simulink model "SistemaUrinario_Simulink"  (R2023a)
settings: Solver=ode15s  StartTime=0.0  StopTime=10.0  RelTol=1e-3
libraries: slpidlib x1
settings Model: Creator=maria  LastModifiedBy=maria
settings DataIOCC: ReturnWorkspaceOutputs=off  TimeSaveName=t
settings DebuggingCC: AlgebraicLoopMsg=none  ArtificialAlgebraicLoopMsg=none  MaxConsecutiveZCsMsg=none  ModelReferenceExtraNoncontSigs=none  OperatingPointInterfaceChecksumMismatchMsg=none

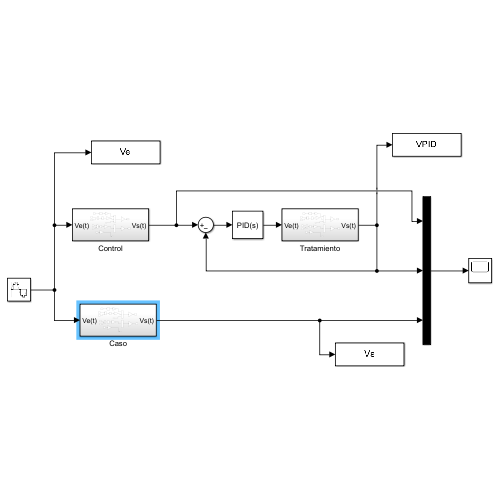
[thumbnail: Simulink's stored preview of the top-level diagram]
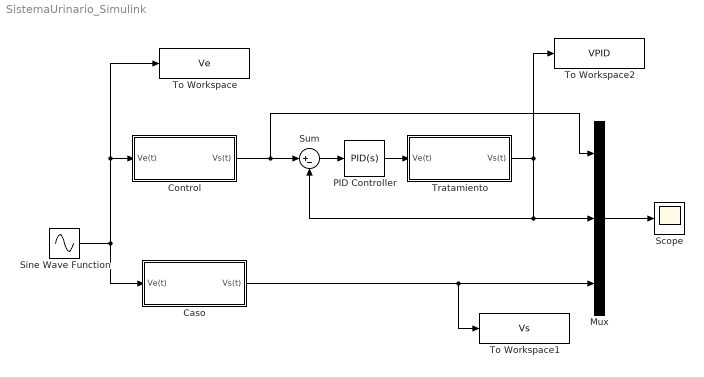
== system SistemaUrinario_Simulink ==
  Caso : Subsystem
  Control : Subsystem
  Mux : Mux  Inputs=3
  PID Controller : slpidlib/PID Controller  Controller=PID  Form=Parallel  TimeDomain=Continuous-time  UseExternalTs=off  SampleTime=-1  IntegratorMethod=Forward Euler  FilterMethod=Forward Euler  ControllerParametersSource=internal  P=8009847.10025754  I=198556446.374402  UseKiTs=off  D=40297.8764782752  N=86.9358796207791  UseFilter=on  TunerSelectOption=Transfer Function Based (PID Tuner App)  InitialConditionSource=internal  InitialConditionForIntegrator=0  InitialConditionForFilter=0  DifferentiatorICPrevScaledInput=0  ExternalReset=none  TrackingMode=off  Kt=1  LimitOutput=off  SatLimitsSource=internal  UpperSaturationLimit=inf  LowerSaturationLimit=-inf  LinearizeAsGain=on  AntiWindupMode=none  Kb=1  LimitIntegrator=off  UpperIntegratorSaturationLimit=inf  LowerIntegratorSaturationLimit=-inf  POutMin=[]  POutMax=[]  IOutMin=[]  IOutMax=[]  DOutMin=[]  DOutMax=[]  NOutMin=[]  NOutMax=[]  SumOutMin=[]  SumOutMax=[]  SaturationOutMin=[]  SaturationOutMax=[]  PParamMin=[]  PParamMax=[]  IParamMin=[]  IParamMax=[]  DParamMin=[]  DParamMax=[]  NParamMin=[]  NParamMax=[]  KbParamMin=[]  KbParamMax=[]  KtParamMin=[]  KtParamMax=[]  KbOutMin=[]  KbOutMax=[]  KtOutMin=[]  KtOutMax=[]  IntegratorOutMin=[]  IntegratorOutMax=[]  FilterOutMin=[]  FilterOutMax=[]  SumI1OutMin=[]  SumI1OutMax=[]  SumI2OutMin=[]  SumI2OutMax=[]  SumI3OutMin=[]  SumI3OutMax=[]  SumI4OutMin=[]  SumI4OutMax=[]  SumDOutMin=[]  SumDOutMax=[]  DifferentiatorOutMin=[]  DifferentiatorOutMax=[]  FilterDiffOutCoefMin=[]  FilterDiffOutCoefMax=[]  ReciprocalOutMin=[]  ReciprocalOutMax=[]  SumDenOutMin=[]  SumDenOutMax=[]  SumNumOutMin=[]  SumNumOutMax=[]  DivideOutMin=[]  DivideOutMax=[]  UdiffTsProdOutMin=[]  UdiffTsProdOutMax=[]  NTsProdOutMin=[]  NTsProdOutMax=[]  UintegralTsProdOutMin=[]  UintegralTsProdOutMax=[]  UngainTsProdOutMin=[]  UngainTsProdOutMax=[]  ClampingZeroOutDataTypeStr=Inherit: Inherit via back propagation  ClampingZeroOutMin=[]  ClampingZeroOutMax=[]  FilterDenConstantOutDataTypeStr=Inherit: Inherit via back propagation  FilterDenConstantOutMin=[]  FilterDenConstantOutMax=[]  PCopyOutDataTypeStr=Inherit: Inherit via back propagation  PCopyOutMin=[]  PCopyOutMax=[]  NCopyOutDataTypeStr=Inherit: Inherit via back propagation  NCopyOutMin=[]  NCopyOutMax=[]  IntegratorContinuousStateAttributes=''  IntegratorStateMustResolveToSignalObject=off  IntegratorRTWStateStorageClass=Auto  FilterContinuousStateAttributes=''  FilterStateMustResolveToSignalObject=off  FilterRTWStateStorageClass=Auto  ParallelPVariant=InternalParameters  IdealPVariant=Disabled  IVariant=InternalParameters  DVariant=InternalParameters  IntegratorVariant=Continuous  SatVariant=Disabled  AWVariant=Passthrough  PCopyVariant=Disabled  TRVariant=Disabled  FdbkBlocksVariant=Forward  IdealPFdbkVariant=Disabled  SatFdbkVariant=Disabled  DerivativeFilterVariant=ContFilter  NVariant=InternalParameters  NCopyVariant=Disabled  FilterICVariant=InternalICsFilter  IntegratorICVariant=InternalICs  ExternalResetVariant=Disabled  TRSumVariant=Passthrough  SumFdbkVariant=Disabled  SumVariant=Sum_PID  TsampFilterVariant=InternalTs  TsampNgainVariant=Passthrough  TsampIntegralVariant=Disabled_SignalSpec  ExternalSaturationOutDataTypeStr=Inherit: Same as second input
  Scope : Scope
  Sine Wave Function : Sin  Frequency=1.5708  SampleTime=0.001
  Sum : Sum  Inputs=|+-
  To Workspace : ToWorkspace  VariableName=Ve  SampleTime=-1
  To Workspace1 : ToWorkspace  VariableName=Vs  SampleTime=-1
  To Workspace2 : ToWorkspace  VariableName=VPID  SampleTime=-1
  Tratamiento : Subsystem
  wires:
  Mux/1 -> Scope/1
  Sine Wave Function/1 -> Caso/1(Ve(t)), To Workspace/1, Control/1(Ve(t))
  Sum/1 -> PID Controller/1
  Control/1(Vs(t)) -> Sum/1, Mux/1
  PID Controller/1 -> Tratamiento/1(Ve(t))
  Caso/1(Vs(t)) -> To Workspace1/1, Mux/3
  Tratamiento/1(Vs(t)) -> Sum/2, Mux/2, To Workspace2/1

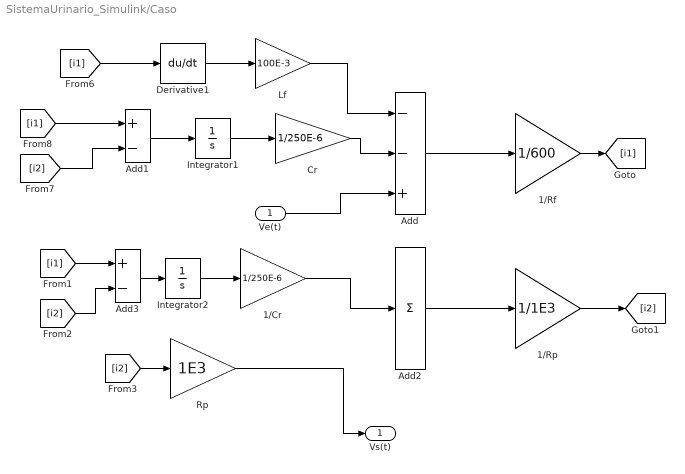
== system SistemaUrinario_Simulink/Caso ==
  Ve(t) : Inport
  1/Cr : Gain  Gain=1/250E-6
  1/Rf : Gain  Gain=1/600
  1/Rp : Gain  Gain=1/1E3
  Add : Sum  Inputs=--+
  Add1 : Sum  Inputs=+-
  Add2 : Sum  Inputs=+
  Add3 : Sum  Inputs=+-
  Cr : Gain  Gain=1/250E-6
  Derivative1 : Derivative
  Integrator1 : Integrator
  Integrator2 : Integrator
  Lf : Gain  Gain=100E-3
  Rp : Gain  Gain=1E3
  Vs(t) : Outport
  wires:
  1/Rp/1 -> [i2]
  [i2] -> Add3/2
  [i2] -> Rp/1
  Add3/1 -> Integrator2/1
  [i1] -> Add3/1
  [i1] -> Add1/1
  [i2] -> Add1/2
  [i1] -> Derivative1/1
  1/Rf/1 -> [i1]
  Add1/1 -> Integrator1/1
  Ve(t)/1 -> Add/3
  Integrator2/1 -> 1/Cr/1
  1/Cr/1 -> Add2/1
  Integrator1/1 -> Cr/1
  Lf/1 -> Add/1
  Derivative1/1 -> Lf/1
  Cr/1 -> Add/2
  Add2/1 -> 1/Rp/1
  Add/1 -> 1/Rf/1
  Rp/1 -> Vs(t)/1

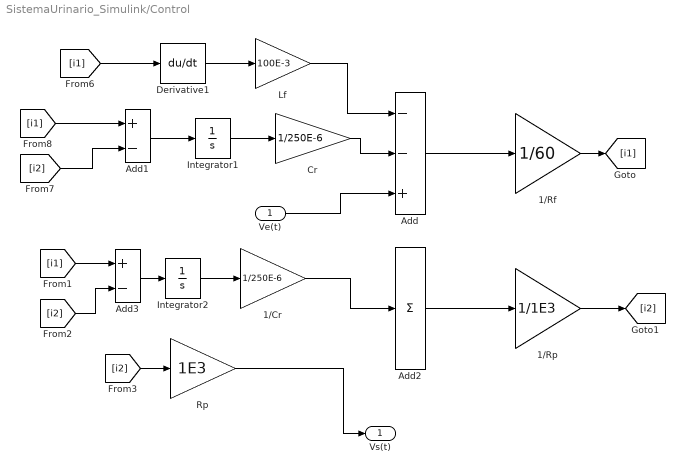
== system SistemaUrinario_Simulink/Control ==
  Ve(t) : Inport
  1/Cr : Gain  Gain=1/250E-6
  1/Rf : Gain  Gain=1/60
  1/Rp : Gain  Gain=1/1E3
  Add : Sum  Inputs=--+
  Add1 : Sum  Inputs=+-
  Add2 : Sum  Inputs=+
  Add3 : Sum  Inputs=+-
  Cr : Gain  Gain=1/250E-6
  Derivative1 : Derivative
  Integrator1 : Integrator
  Integrator2 : Integrator
  Lf : Gain  Gain=100E-3
  Rp : Gain  Gain=1E3
  Vs(t) : Outport
  wires:
  Add/1 -> 1/Rf/1
  Add2/1 -> 1/Rp/1
  Derivative1/1 -> Lf/1
  Lf/1 -> Add/1
  Cr/1 -> Add/2
  Integrator1/1 -> Cr/1
  1/Cr/1 -> Add2/1
  Rp/1 -> Vs(t)/1
  Integrator2/1 -> 1/Cr/1
  Ve(t)/1 -> Add/3
  Add1/1 -> Integrator1/1
  [i1] -> Derivative1/1
  [i2] -> Add1/2
  [i1] -> Add1/1
  Add3/1 -> Integrator2/1
  [i1] -> Add3/1
  [i2] -> Add3/2
  [i2] -> Rp/1
  1/Rf/1 -> [i1]
  1/Rp/1 -> [i2]

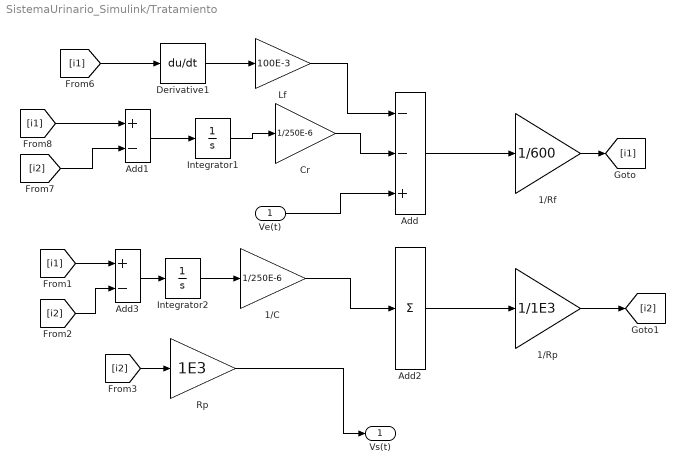
== system SistemaUrinario_Simulink/Tratamiento ==
  Ve(t) : Inport
  1/C : Gain  Gain=1/250E-6
  1/Rf : Gain  Gain=1/600
  1/Rp : Gain  Gain=1/1E3
  Add : Sum  Inputs=--+
  Add1 : Sum  Inputs=+-
  Add2 : Sum  Inputs=+
  Add3 : Sum  Inputs=+-
  Cr : Gain  Gain=1/250E-6
  Derivative1 : Derivative
  Integrator1 : Integrator
  Integrator2 : Integrator
  Lf : Gain  Gain=100E-3
  Rp : Gain  Gain=1E3
  Vs(t) : Outport
  wires:
  1/Rp/1 -> [i2]
  [i2] -> Add3/2
  [i2] -> Rp/1
  Add3/1 -> Integrator2/1
  [i1] -> Add3/1
  [i1] -> Add1/1
  [i2] -> Add1/2
  [i1] -> Derivative1/1
  1/Rf/1 -> [i1]
  Add1/1 -> Integrator1/1
  Ve(t)/1 -> Add/3
  Integrator2/1 -> 1/C/1
  1/C/1 -> Add2/1
  Integrator1/1 -> Cr/1
  Lf/1 -> Add/1
  Derivative1/1 -> Lf/1
  Cr/1 -> Add/2
  Add2/1 -> 1/Rp/1
  Add/1 -> 1/Rf/1
  Rp/1 -> Vs(t)/1
